simulink model "Problem_7_Subsystem"  (R2020b)
settings: Solver=VariableStepAuto  StartTime=0.0  StopTime=10.0  RelTol=1e-3
settings Model: Creator=Yeshwanth  LastModifiedBy=Yeshwanth
settings DataIOCC: SaveOutput=off  SaveTime=off

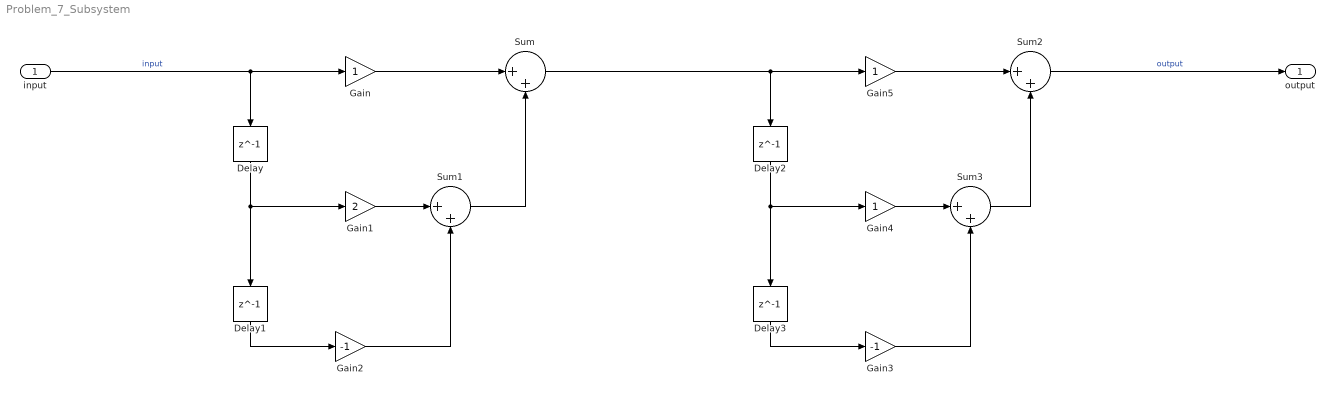
== system Problem_7_Subsystem ==
  input : Inport  OutDataTypeStr=double  PortDimensions=1  SampleTime=0
  Delay{,1..3} (4 alike) : Delay  DelayLength=1
  Gain : Gain
  Gain1 : Gain  Gain=2
  Gain2 : Gain  Gain=-1
  Gain3 : Gain  Gain=-1
  Gain4 : Gain
  Gain5 : Gain
  Sum{,1..3} (4 alike) : Sum  Inputs=|++
  output : Outport  OutDataTypeStr=double  PortDimensions=1  SampleTime=0
  wires:
  Delay/1 -> Delay1/1, Gain1/1
  Delay2/1 -> Delay3/1, Gain4/1
  Sum1/1 -> Sum/2
  Sum/1 -> Delay2/1, Gain5/1
  Gain/1 -> Sum/1
  Gain3/1 -> Sum3/2
  input/1 -> Delay/1, Gain/1  "input"
  Gain1/1 -> Sum1/1
  Delay3/1 -> Gain3/1
  Sum2/1 -> output/1  "output"
  Gain5/1 -> Sum2/1
  Gain4/1 -> Sum3/1
  Sum3/1 -> Sum2/2
  Gain2/1 -> Sum1/2
  Delay1/1 -> Gain2/1
